simulink model "series_shunt_2a"  (Simulink 7.4)
settings: Solver=ode23tb  StartTime=0.0  StopTime=100e-6  MaxStep=10e-9  RelTol=1e-4
InitFcn:
  | series_shunt_2c;
StopFcn:
  | if ~SPECTRUM_FLAG
  |      %% plot measured sparameters using RFTB
  |     amp=rfdata.data;
  |     amp.Freq=spar(:,1);
  | %%
  |     amp.S_parameters=complex(zeros(2,2,length(amp.Freq)));
  |    if spar(1,6)==1
  |       amp.S_Parameters(1,1,:)=spar(:,2)+1i*spar(:,3);
  |       amp.S_Parameters(2,1,:)=spar(:,4)+1i*spar(:,5);
  |       subplot(2,1,1);
  |       hplot1= smith(amp,'s11')
  |       subplot(2,1,2);
  |       hplot2 = plot(amp,'s21');
  |       axis([amp.Freq(1)/1e6,amp.Freq(end)/1e6,0,20]);
  |    else
  |       amp.S_Parameters(2,2,:)=spar(:,2)+1i*spar(:,3);
  |       amp.S_Parameters(1,2,:)=spar(:,4)+1i*spar(:,5);
  |       subplot(2,1,1);
  |       hplot1= smith(amp,'s22')
  |       subplot(2,1,2);
  |       hplot2 = plot(amp,'s12');
  |    end;
  | end
values from neighbouring files (symbols this model uses):
  Base_Bias = 0.8    [series_shunt_2c.m]
  Beta = 100    [series_shunt_2c.m]
  Cbc = 10e-12    (= 1e-11)    [series_shunt_2c.m]
  Cbe = 250e-12    (= 2.5e-10)    [series_shunt_2c.m]
  ICs = IEs    (= 1e-12)    [series_shunt_2c.m]
  IEs = 1e-12    [series_shunt_2c.m]
  Lpri_1 = 5e-6    (= 5e-06)    [series_shunt_2c.m]
  Lsec_1 = Lpri_1*Tr_1^2    [series_shunt_2c.m]
  M12_1 = K*Tr_1*Lpri_1    [series_shunt_2c.m]
  M13_1 = M12_1    [series_shunt_2c.m]
  M23_1 = K*Lsec_1    [series_shunt_2c.m]
  Rbb = 5    [series_shunt_2c.m]
  Re = (Rl^2)/Rfb    (= 1.52007654004)    [series_shunt_2c.m]
  Rfb = Rl*(1*Av+1)    (= 81.21748272)    [series_shunt_2c.m]
  Rloss = .1    (= 0.1)    [series_shunt_2c.m]
  Vcc = 12    [series_shunt_2c.m]
undefined symbols (not defined in the file or in its folder): Fs, magnitude, One, sided
libraries: powerlib x52, dspindex x12, dspsigops x6, dsparch4 x5, simulink x4, dspbuff3 x4, dspxfrm3 x4, dsparch3 x4, dspsnks4 x3, dspmtrx3 x2
(part 1 of 2)
settings Model: Creator=Dick  LastModifiedBy=Dick

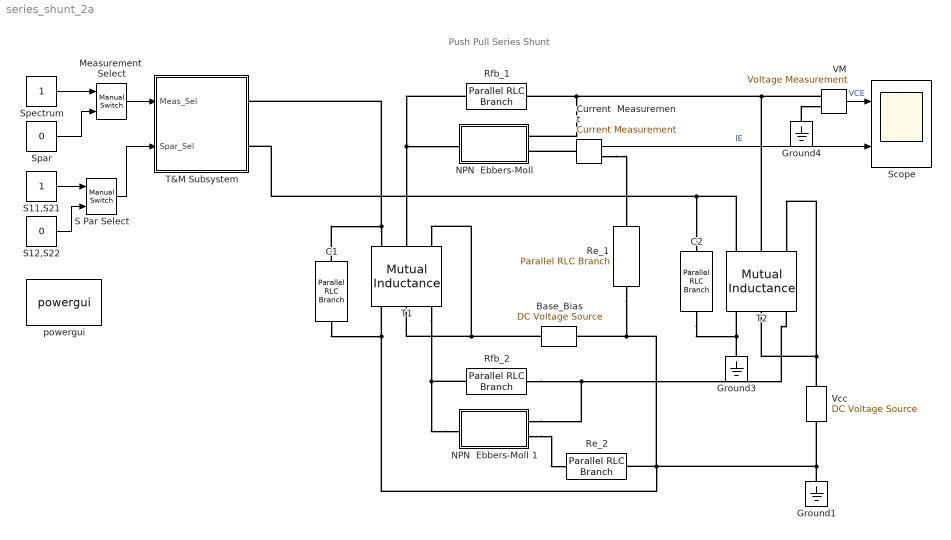
== system series_shunt_2a ==
  note: Push Pull Series Shunt
  Base_Bias : powerlib/Electrical Sources/DC Voltage Source  DialogController=POWERSYS.PowerSysDialog  SystemSampleTime=-1  Amplitude=Base_Bias  Measurements=None
  C1 : powerlib/Elements/Parallel RLC Branch  DialogController=POWERSYS.PowerSysDialog  PhysicalDomain=powersysdomain  SubClassName=unknown  LeftPortType=p1  RightPortType=p1  LConnTagsString=a  RConnTagsString=__new0  BranchType=C  Resistance=1  Inductance=1e-3  SetiL0=off  InitialCurrent=0  Capacitance=2.7e-12  Setx0=off  InitialVoltage=0  Measurements=None
  C2 : powerlib/Elements/Parallel RLC Branch  DialogController=POWERSYS.PowerSysDialog  PhysicalDomain=powersysdomain  SubClassName=unknown  LeftPortType=p1  RightPortType=p1  LConnTagsString=a  RConnTagsString=__new0  BranchType=C  Resistance=1  Inductance=1e-3  SetiL0=off  InitialCurrent=0  Capacitance=27e-12  Setx0=off  InitialVoltage=0  Measurements=None
  Current  Measurement : powerlib/Measurements/Current Measurement  DialogController=POWERSYS.PowerSysDialog  SystemSampleTime=-1  PhasorSimulation=off  OutputType=Complex  PSBequivalent=0
  Ground1 : powerlib/Elements/Ground  DialogController=POWERSYS.PowerSysDialog  PhysicalDomain=powersysdomain  SubClassName=unknown  LeftPortType=p1  RightPortType=p1  LConnTagsString=a
  Ground3 : powerlib/Elements/Ground  DialogController=POWERSYS.PowerSysDialog  PhysicalDomain=powersysdomain  SubClassName=unknown  LeftPortType=p1  RightPortType=p1  LConnTagsString=a
  Ground4 : powerlib/Elements/Ground  DialogController=POWERSYS.PowerSysDialog  PhysicalDomain=powersysdomain  SubClassName=unknown  LeftPortType=p1  RightPortType=p1  LConnTagsString=a
  Measurement  Select : simulink/Signal Routing/Manual Switch  SystemSampleTime=-1  sw=0  action=0  varsize=off
  "NPN  Ebbers-Moll " : Subsystem  mask{Beta=Beta, IEs=IEs, ICs=ICs, Ro=1e5, Cbc=Cbc, Cbe=Cbe, Rbb=Rbb}
      mask init:
      | k = 1.38e-23;
      | q = 1.6e-19;
      | T = 290;
      | Vt = k*T/q;
  NPN  Ebbers-Moll 1 : Subsystem  mask{Beta=Beta, IEs=IEs, ICs=ICs, Ro=1e5, Cbc=Cbc, Cbe=Cbe, Rbb=Rbb}
      mask init:
      | k = 1.38e-23;
      | q = 1.6e-19;
      | T = 290;
      | Vt = k*T/q;
  Re_1 : powerlib/Elements/Parallel RLC Branch  DialogController=POWERSYS.PowerSysDialog  PhysicalDomain=powersysdomain  SubClassName=unknown  LeftPortType=p1  RightPortType=p1  LConnTagsString=a  RConnTagsString=__new0  BranchType=R  Resistance=Re  Inductance=1e-3  SetiL0=off  InitialCurrent=0  Capacitance=1e-6  Setx0=off  InitialVoltage=0  Measurements=None
  Re_2 : powerlib/Elements/Parallel RLC Branch  DialogController=POWERSYS.PowerSysDialog  PhysicalDomain=powersysdomain  SubClassName=unknown  LeftPortType=p1  RightPortType=p1  LConnTagsString=a  RConnTagsString=__new0  BranchType=R  Resistance=Re  Inductance=1e-3  SetiL0=off  InitialCurrent=0  Capacitance=1e-6  Setx0=off  InitialVoltage=0  Measurements=None
  Rfb_1 : powerlib/Elements/Parallel RLC Branch  DialogController=POWERSYS.PowerSysDialog  PhysicalDomain=powersysdomain  SubClassName=unknown  LeftPortType=p1  RightPortType=p1  LConnTagsString=a  RConnTagsString=__new0  BranchType=R  Resistance=Rfb  Inductance=1e-3  SetiL0=off  InitialCurrent=0  Capacitance=1e-6  Setx0=off  InitialVoltage=0  Measurements=None
  Rfb_2 : powerlib/Elements/Parallel RLC Branch  DialogController=POWERSYS.PowerSysDialog  PhysicalDomain=powersysdomain  SubClassName=unknown  LeftPortType=p1  RightPortType=p1  LConnTagsString=a  RConnTagsString=__new0  BranchType=R  Resistance=Rfb  Inductance=1e-3  SetiL0=off  InitialCurrent=0  Capacitance=1e-6  Setx0=off  InitialVoltage=0  Measurements=None
  S Par Select : simulink/Signal Routing/Manual Switch  SystemSampleTime=-1  sw=1  action=0  varsize=off
  S11,S21 : Constant  OutDataType=fixdt(1, 16)  OutScaling=2^0
  S12,S22 : Constant  Value=0  OutDataType=fixdt(1, 16)  OutScaling=2^0
  Scope : Scope  NumInputPorts=2
      settings: TimeRange=5e-006  YMin=-17.5~-0.1  YMax=17.5~1.5
  Spar : Constant  Value=0  OutDataTypeMode=boolean  OutDataType=fixdt(1, 16)  OutScaling=2^0  OutDataTypeStr=boolean
  Spectrum : Constant  OutDataTypeMode=boolean  OutDataType=fixdt(1, 16)  OutScaling=2^0  OutDataTypeStr=boolean
  T&M Subsystem : Subsystem
  T1 : powerlib/Elements/Mutual Inductance  DialogController=POWERSYS.PowerSysDialog  PhysicalDomain=powersysdomain  SubClassName=unknown  LeftPortType=p1  RightPortType=p1  LConnTagsString=a|b|c  RConnTagsString=A|B|C  TypeOfMutual=Generalized mutual inductance  NumberOfWindings=3  SelfImpedance1=[1.1 1.1e-03]  SelfImpedance2=[ 1.1 1.1e-03]  ThreeWindings=on  SelfImpedance3=[ 1.1 1.1e-03]  MutualImpedance=[1.0 1.0e-03]  InductanceMatrix=[Lpri_1 M12_1 M13_1; M12_1 Lsec_1 M23_1; M13_1 M23_1 Lsec_1];  ResistanceMatrix="[1  0 0 ; 0 1 0 ; 0 0 1]*Rloss;"  Measurements=None
      settings: AttributesFormatString=\n
  T2 : powerlib/Elements/Mutual Inductance  DialogController=POWERSYS.PowerSysDialog  PhysicalDomain=powersysdomain  SubClassName=unknown  LeftPortType=p1  RightPortType=p1  LConnTagsString=a|b|c  RConnTagsString=A|B|C  TypeOfMutual=Generalized mutual inductance  NumberOfWindings=3  SelfImpedance1=[1.1 1.1e-03]  SelfImpedance2=[ 1.1 1.1e-03]  ThreeWindings=on  SelfImpedance3=[ 1.1 1.1e-03]  MutualImpedance=[1.0 1.0e-03]  InductanceMatrix=[Lpri_1 M12_1 M13_1; M12_1 Lsec_1 M23_1; M13_1 M23_1 Lsec_1];  ResistanceMatrix="[1  0 0 ; 0 1 0 ; 0 0 1]*Rloss;"  Measurements=None
      settings: AttributesFormatString=\n
  VM : powerlib/Measurements/Voltage Measurement  DialogController=POWERSYS.PowerSysDialog  SystemSampleTime=-1  PhasorSimulation=off  OutputType=Complex  PSBequivalent=0
  Vcc : powerlib/Electrical Sources/DC Voltage Source  DialogController=POWERSYS.PowerSysDialog  SystemSampleTime=-1  Amplitude=Vcc  Measurements=None
  powergui : powerlib/powergui  Priority=1  SystemSampleTime=-1  SimulationMode=Continuous  SampleTime=50e-6  frequency=60  SPID=off  DisableSnubberDevices=off  DisableRonSwitches=off  DisableVfSwitches=off  SwTol=0  Interpol=off  frequencyindice=0  echomessages=off  HookPort=off  DisplayEquations=off  FunctionMessages=off  EnableUseOfTLC=off  x0status=blocks  RestoreLinks=warning  Frange=[0:2:500]  Ylog=off  Xlog=on  ShowGrid=off  save=off  variable=ZData  ZoomFFT=on  StartTime=0.0  cycles=1  DisplayStyle=1  fundamental=60  FreqAxis=off  MaxFrequency=1000  frequencyindicesteady=1  RmsSteady=1  display=off  Ts=0  methode=off
  wires:
  Measurement  Select/1 -> T&M Subsystem/1(Meas_Sel)
  Spar/1 -> Measurement  Select/2
  Spectrum/1 -> Measurement  Select/1
  S Par Select/1 -> T&M Subsystem/2(Spar_Sel)
  S11,S21/1 -> S Par Select/1
  S12,S22/1 -> S Par Select/2
  VM/1 -> Scope/1  "VCE"
  Current  Measurement/1 -> Scope/2  "IE"
  connections:
  VM/LConn1 -- Rfb_1/LConn1 -- "NPN  Ebbers-Moll "/RConn1 -- T2/RConn2
  Rfb_1/RConn1 -- T1/RConn2 -- "NPN  Ebbers-Moll "/LConn1
  Base_Bias/LConn1 -- Re_1/RConn1 -- Re_2/LConn1 -- Ground1/LConn1 -- Vcc/LConn1 -- T1/LConn1 -- C1/RConn1
  T1/RConn1 -- C1/LConn1 -- T&M Subsystem/RConn1
  T2/RConn1 -- T&M Subsystem/RConn2 -- C2/LConn1
  Current  Measurement/LConn1 -- "NPN  Ebbers-Moll "/RConn2
  Current  Measurement/RConn1 -- Re_1/LConn1
  Vcc/RConn1 -- T2/RConn3 -- T2/LConn2
  Ground3/LConn1 -- T2/LConn1 -- C2/RConn1
  T1/LConn2 -- Base_Bias/RConn1 -- T1/RConn3
  NPN  Ebbers-Moll 1/LConn1 -- T1/LConn3 -- Rfb_2/RConn1
  Rfb_2/LConn1 -- T2/LConn3 -- NPN  Ebbers-Moll 1/RConn1
  Ground4/LConn1 -- VM/LConn2
  NPN  Ebbers-Moll 1/RConn2 -- Re_2/RConn1

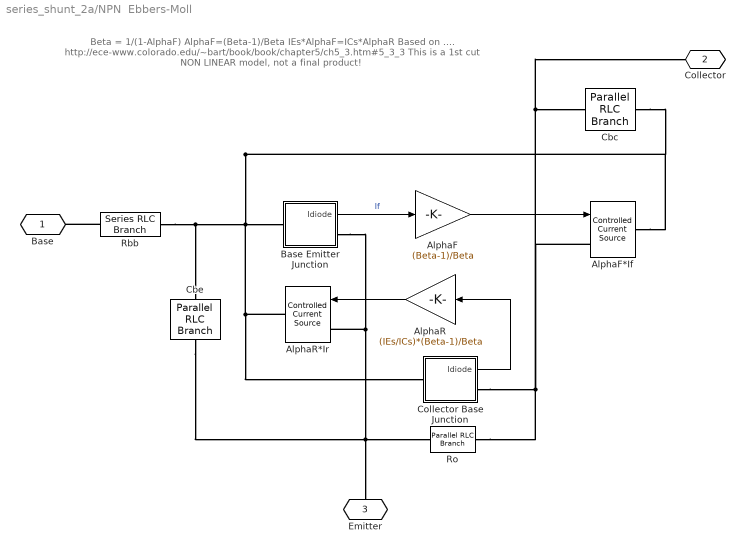
== system series_shunt_2a/NPN  Ebbers-Moll  ==
  note: Beta = 1/(1-AlphaF)
      | AlphaF=(Beta-1)/Beta
      | IEs*AlphaF=ICs*AlphaR
      |
      | Based on ....
      | http://ece-www.colorado.edu/~bart/book/book/chapter5/ch5_3.htm#5_3_3
      |
      | This is a 1st cut NON LINEAR model, not a final product!
  AlphaF : Gain  Gain=(Beta-1)/Beta  ParameterDataType=sfix(16)  ParameterScaling=2^0  OutDataType=sfix(16)  OutScaling=2^0
  AlphaF*If : powerlib/Electrical Sources/Controlled Current Source  Description=source block  DialogController=POWERSYS.PowerSysDialog  SystemSampleTime=-1  Initialize=off  Source_Type=AC  Amplitude=-0.025  Phase=0  Frequency=0  Measurements=None
      settings: AttributesFormatString=\n
  AlphaR : Gain  Gain=(IEs/ICs)*(Beta-1)/Beta  ParameterDataType=sfix(16)  ParameterScaling=2^0  OutDataType=sfix(16)  OutScaling=2^0
  AlphaR*Ir : powerlib/Electrical Sources/Controlled Current Source  Description=source block  DialogController=POWERSYS.PowerSysDialog  SystemSampleTime=-1  Initialize=off  Source_Type=AC  Amplitude=-0.025  Phase=0  Frequency=0  Measurements=None
      settings: AttributesFormatString=\n
  Base Emitter Junction : Subsystem  AncestorBlock=simcircuits_library_1/diode  mask{Is=IEs}
      mask prompts: Is "Saturation Current"
      mask Display: plot(-140,-140,150,140,2*[30,30,59,30,30,0]-75,(2*[71,50,72,92,71,71]-92),2*[59,59]-75,(2*[50,93]-92),[116,59]-16,(2*[71,71]-90));
  Cbc : powerlib/Elements/Parallel RLC Branch  DialogController=POWERSYS.PowerSysDialog  PhysicalDomain=powersysdomain  SubClassName=unknown  LeftPortType=p1  RightPortType=p1  LConnTagsString=a  RConnTagsString=__new0  BranchType=C  Resistance=1.0  Inductance=1.0  SetiL0=off  InitialCurrent=0  Capacitance=Cbc  Setx0=off  InitialVoltage=0  Measurements=None
  Cbe : powerlib/Elements/Parallel RLC Branch  DialogController=POWERSYS.PowerSysDialog  PhysicalDomain=powersysdomain  SubClassName=unknown  LeftPortType=p1  RightPortType=p1  LConnTagsString=a  RConnTagsString=__new0  BranchType=C  Resistance=1.0  Inductance=1.0  SetiL0=off  InitialCurrent=0  Capacitance=Cbe  Setx0=off  InitialVoltage=0  Measurements=None
  Collector Base Junction : Subsystem  AncestorBlock=simcircuits_library_1/diode  mask{Is=ICs}
      mask prompts: Is "Saturation Current"
      mask Display: plot(-140,-140,150,140,2*[30,30,59,30,30,0]-75,(2*[71,50,72,92,71,71]-92),2*[59,59]-75,(2*[50,93]-92),[116,59]-16,(2*[71,71]-90));
  Rbb : powerlib/Elements/Series RLC Branch  DialogController=POWERSYS.PowerSysDialog  PhysicalDomain=powersysdomain  SubClassName=unknown  LeftPortType=p1  RightPortType=p1  LConnTagsString=__new0  RConnTagsString=__new0  BranchType=R  Resistance=Rbb  Inductance=1.0  SetiL0=off  InitialCurrent=0  Capacitance=1.0  Setx0=off  InitialVoltage=0  Measurements=None
  Ro : powerlib/Elements/Parallel RLC Branch  DialogController=POWERSYS.PowerSysDialog  PhysicalDomain=powersysdomain  SubClassName=unknown  LeftPortType=p1  RightPortType=p1  LConnTagsString=a  RConnTagsString=__new0  BranchType=R  Resistance=Ro  Inductance=1.0  SetiL0=off  InitialCurrent=0  Capacitance=1.0  Setx0=off  InitialVoltage=0  Measurements=None
  Base : PMIOPort  Port=1  Side=Left
  Collector : PMIOPort  Port=2  Side=Right
  Emitter : PMIOPort  Port=3  Side=Right
  wires:
  Base Emitter Junction/1(Idiode) -> AlphaF/1  "If"
  AlphaF/1 -> AlphaF*If/1
  Collector Base Junction/1(Idiode) -> AlphaR/1
  AlphaR/1 -> AlphaR*Ir/1
  connections:
  Rbb/RConn1 -- Cbe/LConn1 -- Base Emitter Junction/LConn1 -- AlphaF*If/RConn1 -- Cbc/RConn1 -- AlphaR*Ir/RConn1 -- Collector Base Junction/LConn1
  AlphaR*Ir/LConn1 -- Emitter/RConn1 -- Cbe/RConn1 -- Ro/LConn1 -- Base Emitter Junction/RConn1
  AlphaF*If/LConn1 -- Collector/RConn1 -- Cbc/LConn1 -- Collector Base Junction/RConn1 -- Ro/RConn1
  Rbb/LConn1 -- Base/RConn1

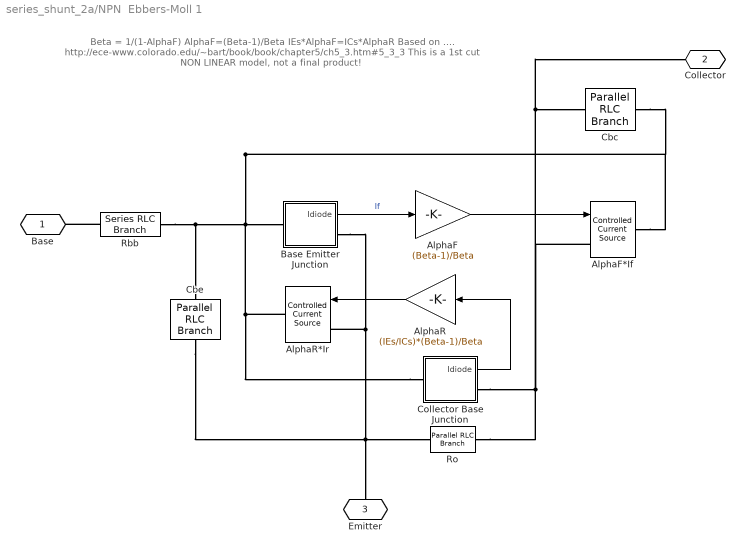
== system series_shunt_2a/NPN  Ebbers-Moll 1 ==
  note: Beta = 1/(1-AlphaF)
      | AlphaF=(Beta-1)/Beta
      | IEs*AlphaF=ICs*AlphaR
      |
      | Based on ....
      | http://ece-www.colorado.edu/~bart/book/book/chapter5/ch5_3.htm#5_3_3
      |
      | This is a 1st cut NON LINEAR model, not a final product!
  AlphaF : Gain  Gain=(Beta-1)/Beta  ParameterDataType=sfix(16)  ParameterScaling=2^0  OutDataType=sfix(16)  OutScaling=2^0
  AlphaF*If : powerlib/Electrical Sources/Controlled Current Source  Description=source block  DialogController=POWERSYS.PowerSysDialog  SystemSampleTime=-1  Initialize=off  Source_Type=AC  Amplitude=-0.025  Phase=0  Frequency=0  Measurements=None
      settings: AttributesFormatString=\n
  AlphaR : Gain  Gain=(IEs/ICs)*(Beta-1)/Beta  ParameterDataType=sfix(16)  ParameterScaling=2^0  OutDataType=sfix(16)  OutScaling=2^0
  AlphaR*Ir : powerlib/Electrical Sources/Controlled Current Source  Description=source block  DialogController=POWERSYS.PowerSysDialog  SystemSampleTime=-1  Initialize=off  Source_Type=AC  Amplitude=-0.025  Phase=0  Frequency=0  Measurements=None
      settings: AttributesFormatString=\n
  Base Emitter Junction : Subsystem  AncestorBlock=simcircuits_library_1/diode  mask{Is=IEs}
      mask prompts: Is "Saturation Current"
      mask Display: plot(-140,-140,150,140,2*[30,30,59,30,30,0]-75,(2*[71,50,72,92,71,71]-92),2*[59,59]-75,(2*[50,93]-92),[116,59]-16,(2*[71,71]-90));
  Cbc : powerlib/Elements/Parallel RLC Branch  DialogController=POWERSYS.PowerSysDialog  PhysicalDomain=powersysdomain  SubClassName=unknown  LeftPortType=p1  RightPortType=p1  LConnTagsString=a  RConnTagsString=__new0  BranchType=C  Resistance=1.0  Inductance=1.0  SetiL0=off  InitialCurrent=0  Capacitance=Cbc  Setx0=off  InitialVoltage=0  Measurements=None
  Cbe : powerlib/Elements/Parallel RLC Branch  DialogController=POWERSYS.PowerSysDialog  PhysicalDomain=powersysdomain  SubClassName=unknown  LeftPortType=p1  RightPortType=p1  LConnTagsString=a  RConnTagsString=__new0  BranchType=C  Resistance=1.0  Inductance=1.0  SetiL0=off  InitialCurrent=0  Capacitance=Cbe  Setx0=off  InitialVoltage=0  Measurements=None
  Collector Base Junction : Subsystem  AncestorBlock=simcircuits_library_1/diode  mask{Is=ICs}
      mask prompts: Is "Saturation Current"
      mask Display: plot(-140,-140,150,140,2*[30,30,59,30,30,0]-75,(2*[71,50,72,92,71,71]-92),2*[59,59]-75,(2*[50,93]-92),[116,59]-16,(2*[71,71]-90));
  Rbb : powerlib/Elements/Series RLC Branch  DialogController=POWERSYS.PowerSysDialog  PhysicalDomain=powersysdomain  SubClassName=unknown  LeftPortType=p1  RightPortType=p1  LConnTagsString=__new0  RConnTagsString=__new0  BranchType=R  Resistance=Rbb  Inductance=1.0  SetiL0=off  InitialCurrent=0  Capacitance=1.0  Setx0=off  InitialVoltage=0  Measurements=None
  Ro : powerlib/Elements/Parallel RLC Branch  DialogController=POWERSYS.PowerSysDialog  PhysicalDomain=powersysdomain  SubClassName=unknown  LeftPortType=p1  RightPortType=p1  LConnTagsString=a  RConnTagsString=__new0  BranchType=R  Resistance=Ro  Inductance=1.0  SetiL0=off  InitialCurrent=0  Capacitance=1.0  Setx0=off  InitialVoltage=0  Measurements=None
  Base : PMIOPort  Port=1  Side=Left
  Collector : PMIOPort  Port=2  Side=Right
  Emitter : PMIOPort  Port=3  Side=Right
  wires:
  AlphaR/1 -> AlphaR*Ir/1
  Collector Base Junction/1(Idiode) -> AlphaR/1
  AlphaF/1 -> AlphaF*If/1
  Base Emitter Junction/1(Idiode) -> AlphaF/1  "If"
  connections:
  Rbb/LConn1 -- Base/RConn1
  Ro/RConn1 -- Collector Base Junction/RConn1 -- Cbc/LConn1 -- Collector/RConn1 -- AlphaF*If/LConn1
  Base Emitter Junction/RConn1 -- Ro/LConn1 -- Cbe/RConn1 -- Emitter/RConn1 -- AlphaR*Ir/LConn1
  Collector Base Junction/LConn1 -- AlphaR*Ir/RConn1 -- Cbc/RConn1 -- AlphaF*If/RConn1 -- Base Emitter Junction/LConn1 -- Cbe/LConn1 -- Rbb/RConn1

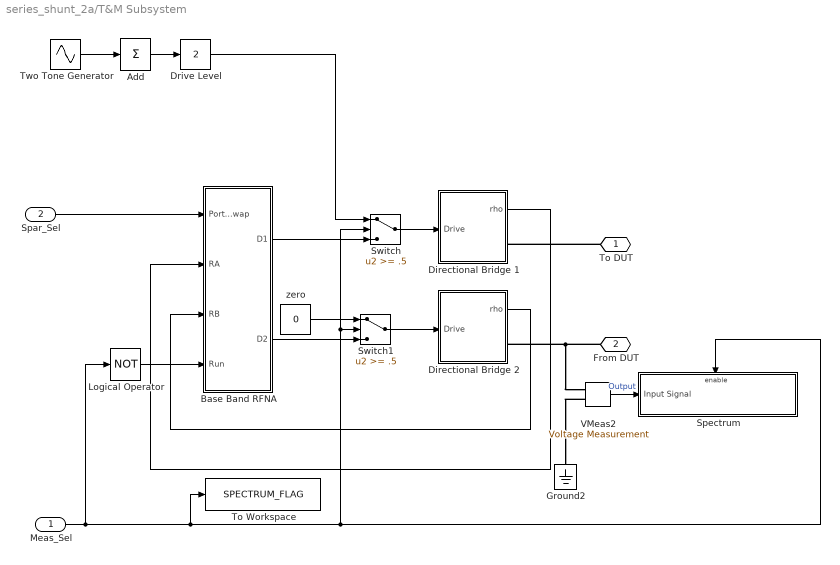
== system series_shunt_2a/T&M Subsystem ==
  Meas_Sel : Inport  OutDataType=fixdt(1, 16)  OutScaling=2^0
  Spar_Sel : Inport  Port=2  OutDataType=fixdt(1, 16)  OutScaling=2^0
  Add : Sum  Inputs=+  OutDataType=fixdt(1, 16)  OutScaling=2^-10
  Base Band RFNA : Subsystem  Description=Spectrum Analyzer  mask{BW=30e6, Frame_Size=256}
      mask prompts: BW "Bandwidth"; Frame_Size "FFT SIze (256,512,1024 etc)"
  Directional Bridge 1 : Subsystem  mask{Zo=50}
      mask prompts: Zo "Zo="
  Directional Bridge 2 : Subsystem  mask{Zo=50}
      mask prompts: Zo "Zo="
  Drive Level : simulink/Math Operations/Slider Gain  SystemSampleTime=-1  low=0.2  gain=2  high=4
  Ground2 : powerlib/Elements/Ground  DialogController=POWERSYS.PowerSysDialog  PhysicalDomain=powersysdomain  SubClassName=unknown  LeftPortType=p1  RightPortType=p1  LConnTagsString=a
  Logical Operator : Logic  Operator=NOT  AllPortsSameDT=off  OutDataTypeMode=boolean  LogicDataType=fixdt(0, 8)  OutDataTypeStr=boolean
  Spectrum : Subsystem  Description=Spectrum Analyzer  mask{BW=30e6, Zo=50}
      mask prompts: BW "Bandwidth"; Zo "Load Zo"
      mask Display: fprintf('Baseband Spectrum Analyzer \n  BW=%7.2f MHz', BW/1e6)
  Switch : Switch  Threshold=.5  OutDataType=fixdt(1, 16)  OutScaling=2^0
  Switch1 : Switch  Threshold=.5  OutDataType=fixdt(1, 16)  OutScaling=2^0
  To Workspace : ToWorkspace  VariableName=SPECTRUM_FLAG  SampleTime=-1  SaveFormat=Array
      settings: MaxDataPoints=1
  Two Tone Generator : Sin  Amplitude=2*sqrt(2)  Bias=0  Frequency=[10e6 12e6]*2*pi  Phase=0  Samples=10  SampleTime=0  Offset=0
  VMeas2 : powerlib/Measurements/Voltage Measurement  DialogController=POWERSYS.PowerSysDialog  SystemSampleTime=-1  PhasorSimulation=off  OutputType=Complex  PSBequivalent=0
  zero : Constant  Value=0  OutDataTypeMode=boolean  OutDataType=fixdt(1, 16)  OutScaling=2^0  OutDataTypeStr=boolean
  To DUT : PMIOPort  Port=1  Side=Right
  From DUT : PMIOPort  Port=2  Side=Right
  wires:
  Two Tone Generator/1 -> Add/1
  Directional Bridge 1/1(rho) -> Base Band RFNA/2(RA)
  Directional Bridge 2/1(rho) -> Base Band RFNA/3(RB)
  VMeas2/1 -> Spectrum/1(Input Signal)  "Output"
  Base Band RFNA/1(D1) -> Switch/3
  Switch/1 -> Directional Bridge 1/1(Drive)
  Add/1 -> Drive Level/1
  Switch1/1 -> Directional Bridge 2/1(Drive)
  Base Band RFNA/2(D2) -> Switch1/3
  zero/1 -> Switch1/1
  Logical Operator/1 -> Base Band RFNA/4(Run)
  Meas_Sel/1 -> Logical Operator/1, Switch1/2, Switch/2, Spectrum/Enable, To Workspace/1
  Spar_Sel/1 -> Base Band RFNA/1(Port Swap)
  Drive Level/1 -> Switch/1
  connections:
  From DUT/RConn1 -- Directional Bridge 2/RConn1 -- VMeas2/LConn1
  VMeas2/LConn2 -- Ground2/LConn1
  To DUT/RConn1 -- Directional Bridge 1/RConn1

== system series_shunt_2a/NPN  Ebbers-Moll /Base Emitter Junction ==
  Diode Equation : Fcn  Expr="Is* (exp(u /.025)  -1  );  % ideal diode equation @ room temp"
  "Vf " : powerlib/Measurements/Voltage Measurement  Tag=PoWeRsYsTeMmEaSuReMeNt  DialogController=POWERSYS.PowerSysDialog  SystemSampleTime=-1  PhasorSimulation=off  OutputType=Magnitude  PSBequivalent=0
  ik1 : powerlib/Electrical Sources/Controlled Current Source  Description=source block  DialogController=POWERSYS.PowerSysDialog  SystemSampleTime=-1  Initialize=on  Source_Type=AC  Amplitude=0  Phase=0  Frequency=0  Measurements=None
      settings: AttributesFormatString=\n
  Anode : PMIOPort  Tag=PMCPort  Port=1  Side=Left
  "cathode " : PMIOPort  Tag=PMCPort  Port=2  Side=Right
  Idiode : Outport  OutDataType=sfix(16)  OutScaling=2^0
  wires:
  "Vf "/1 -> Diode Equation/1
  Diode Equation/1 -> ik1/1, Idiode/1
  connections:
  "Vf "/LConn1 -- Anode/RConn1 -- ik1/LConn1
  "Vf "/LConn2 -- "cathode "/RConn1 -- ik1/RConn1

== system series_shunt_2a/NPN  Ebbers-Moll /Collector Base Junction ==
  Diode Equation : Fcn  Expr="Is* (exp(u /.025)  -1  );  % ideal diode equation @ room temp"
  "Vf " : powerlib/Measurements/Voltage Measurement  Tag=PoWeRsYsTeMmEaSuReMeNt  DialogController=POWERSYS.PowerSysDialog  SystemSampleTime=-1  PhasorSimulation=off  OutputType=Magnitude  PSBequivalent=0
  ik1 : powerlib/Electrical Sources/Controlled Current Source  Description=source block  DialogController=POWERSYS.PowerSysDialog  SystemSampleTime=-1  Initialize=on  Source_Type=AC  Amplitude=0  Phase=0  Frequency=0  Measurements=None
      settings: AttributesFormatString=\n
  Anode : PMIOPort  Tag=PMCPort  Port=1  Side=Left
  "cathode " : PMIOPort  Tag=PMCPort  Port=2  Side=Right
  Idiode : Outport  OutDataType=sfix(16)  OutScaling=2^0
  wires:
  Diode Equation/1 -> Idiode/1, ik1/1
  "Vf "/1 -> Diode Equation/1
  connections:
  ik1/RConn1 -- "cathode "/RConn1 -- "Vf "/LConn2
  ik1/LConn1 -- Anode/RConn1 -- "Vf "/LConn1

== system series_shunt_2a/NPN  Ebbers-Moll 1/Base Emitter Junction ==
  Diode Equation : Fcn  Expr="Is* (exp(u /.025)  -1  );  % ideal diode equation @ room temp"
  "Vf " : powerlib/Measurements/Voltage Measurement  Tag=PoWeRsYsTeMmEaSuReMeNt  DialogController=POWERSYS.PowerSysDialog  SystemSampleTime=-1  PhasorSimulation=off  OutputType=Magnitude  PSBequivalent=0
  ik1 : powerlib/Electrical Sources/Controlled Current Source  Description=source block  DialogController=POWERSYS.PowerSysDialog  SystemSampleTime=-1  Initialize=on  Source_Type=AC  Amplitude=0  Phase=0  Frequency=0  Measurements=None
      settings: AttributesFormatString=\n
  Anode : PMIOPort  Tag=PMCPort  Port=1  Side=Left
  "cathode " : PMIOPort  Tag=PMCPort  Port=2  Side=Right
  Idiode : Outport  OutDataType=sfix(16)  OutScaling=2^0
  wires:
  Diode Equation/1 -> Idiode/1, ik1/1
  "Vf "/1 -> Diode Equation/1
  connections:
  ik1/RConn1 -- "cathode "/RConn1 -- "Vf "/LConn2
  ik1/LConn1 -- Anode/RConn1 -- "Vf "/LConn1

== system series_shunt_2a/NPN  Ebbers-Moll 1/Collector Base Junction ==
  Diode Equation : Fcn  Expr="Is* (exp(u /.025)  -1  );  % ideal diode equation @ room temp"
  "Vf " : powerlib/Measurements/Voltage Measurement  Tag=PoWeRsYsTeMmEaSuReMeNt  DialogController=POWERSYS.PowerSysDialog  SystemSampleTime=-1  PhasorSimulation=off  OutputType=Magnitude  PSBequivalent=0
  ik1 : powerlib/Electrical Sources/Controlled Current Source  Description=source block  DialogController=POWERSYS.PowerSysDialog  SystemSampleTime=-1  Initialize=on  Source_Type=AC  Amplitude=0  Phase=0  Frequency=0  Measurements=None
      settings: AttributesFormatString=\n
  Anode : PMIOPort  Tag=PMCPort  Port=1  Side=Left
  "cathode " : PMIOPort  Tag=PMCPort  Port=2  Side=Right
  Idiode : Outport  OutDataType=sfix(16)  OutScaling=2^0
  wires:
  "Vf "/1 -> Diode Equation/1
  Diode Equation/1 -> ik1/1, Idiode/1
  connections:
  "Vf "/LConn1 -- Anode/RConn1 -- ik1/LConn1
  "Vf "/LConn2 -- "cathode "/RConn1 -- ik1/RConn1

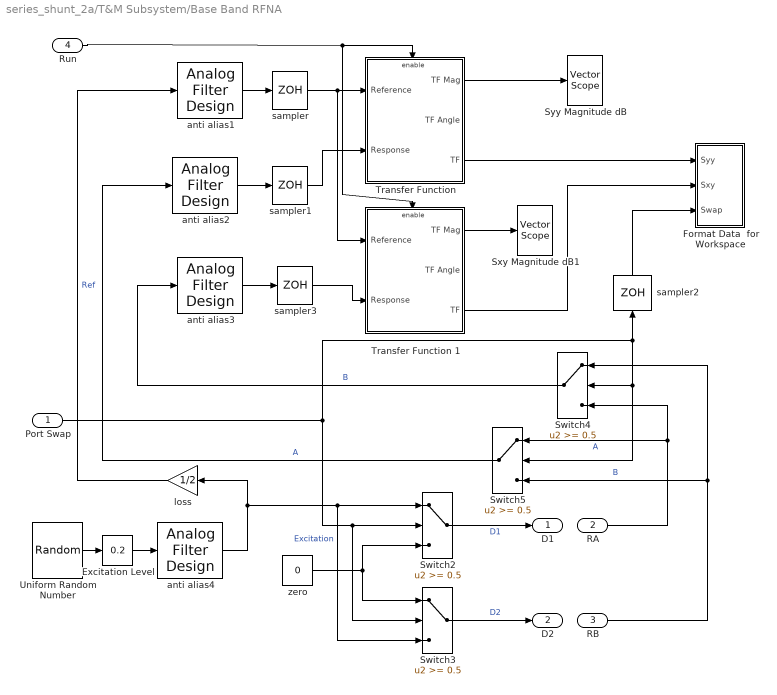
== system series_shunt_2a/T&M Subsystem/Base Band RFNA ==
  Port Swap : Inport  OutDataType=sfix(16)  OutScaling=2^0
  RA : Inport  Port=2  OutDataType=fixdt(1, 16)  OutScaling=2^0
  RB : Inport  Port=3  OutDataType=fixdt(1, 16)  OutScaling=2^0
  Run : Inport  Port=4  OutDataType=sfix(16)  OutScaling=2^0
  Excitation Level : simulink/Math Operations/Slider Gain  SystemSampleTime=-1  low=0  gain=0.2  high=1
  Format Data  for Workspace : Subsystem
  Switch{2..5} (4 alike) : Switch  Threshold=0.5  SaturateOnIntegerOverflow=on
  Sxy Magnitude dB1 : dspsnks4/Vector Scope  DialogController=dspdialog.VectorScope  DialogControllerArgs=DataTag0  ScopeProperties=on  Domain=Frequency  HorizSpan=1  DisplayProperties=off  AxisGrid=on  Memory=off  FrameNumber=on  AxisLegend=off  AxisZoom=off  OpenScopeAtSimStart=on  OpenScopeImmediately=off  FigPos=[414 33 372 236]  AxisProperties=off  XUnits=Hertz  XRange=[0...Fs/2]  InheritXIncr=on  XIncr=2*Fs  XLabel=Time  XLimit=Auto  XMin=0  XMax=1  XStart=0  YUnits=dB  YLabel=dB  LineProperties=off  LineColors=[1 0 0]|[1 0 0]  XAxisParamsVer=6.9
      settings: YMin=0  YMax=25
  Syy Magnitude dB : dspsnks4/Vector Scope  DialogController=dspdialog.VectorScope  DialogControllerArgs=DataTag1  ScopeProperties=on  Domain=Frequency  HorizSpan=1  DisplayProperties=off  AxisGrid=on  Memory=off  FrameNumber=on  AxisLegend=off  AxisZoom=off  OpenScopeAtSimStart=on  OpenScopeImmediately=off  FigPos=[32 34 372 236]  AxisProperties=off  XUnits=Hertz  XRange=[0...Fs/2]  InheritXIncr=on  XIncr=2*Fs  XLabel=Time  XLimit=Auto  XMin=0  XMax=128000000  XStart=0  YUnits=dB  YLabel=dB  LineProperties=off  LineColors=[1 0 0]|[1 0 0]  XAxisParamsVer=6.9
      settings: YMin=-40  YMax=0
  "Transfer Function " : Subsystem  mask{NFFT=Frame_Size, Navg=100, pcnt=100, unwrap_flag=on}
      mask prompts: NFFT "FFT length (power of 2):"; Navg "Spectral Averaging Factor (>=1):"; pcnt "Percentage of  Alias Free Data  (<=100)"; unwrap_flag "Unwrap Phase"
      mask Display: disp('Transfer Function \n Estimation (v2.0) ')
  Transfer Function 1 : Subsystem  mask{NFFT=Frame_Size, Navg=100, pcnt=100, unwrap_flag=on}
      mask prompts: NFFT "FFT length (power of 2):"; Navg "Spectral Averaging Factor (>=1):"; pcnt "Percentage of  Alias Free Data  (<=100)"; unwrap_flag "Unwrap Phase"
      mask Display: disp('Transfer Function \n Estimation (v2.0) ')
  Uniform Random Number : UniformRandomNumber  SampleTime=1/(2.56*BW)
  anti alias{1..4} (4 alike) : dsparch4/Analog Filter Design  method=Elliptic  filttype=Lowpass  N=8  Wlo=BW*2*pi  Whi=80  Rp=2  Rs=100
  loss : Gain  Gain=1/2  ParameterDataType=sfix(16)  ParameterScaling=2^0  OutDataType=sfix(16)  OutScaling=2^0  SaturateOnIntegerOverflow=on  OutDataTypeStr=Inherit: Same as input  ParamDataTypeStr=Inherit: Same as input
  sampler : ZeroOrderHold  SampleTime=1/(2.56*BW)
  sampler1 : ZeroOrderHold  SampleTime=1/(2.56*BW)
  sampler2 : ZeroOrderHold  SampleTime=256/(2.56*BW)
  sampler3 : ZeroOrderHold  SampleTime=1/(2.56*BW)
  zero : Constant  Value=0  OutDataType=sfix(16)  OutScaling=2^0
  D1 : Outport  OutDataType=fixdt(1, 16)  OutScaling=2^0
  D2 : Outport  Port=2  OutDataType=fixdt(1, 16)  OutScaling=2^0
  wires:
  sampler/1 -> "Transfer Function "/1(Reference), Transfer Function 1/1(Reference)
  anti alias1/1 -> sampler/1
  anti alias2/1 -> sampler1/1
  Uniform Random Number/1 -> Excitation Level/1
  anti alias3/1 -> sampler3/1
  sampler3/1 -> Transfer Function 1/2(Response)
  anti alias4/1 -> loss/1, Switch3/3, Switch2/1  "Excitation"
  loss/1 -> anti alias1/1  "Ref"
  Port Swap/1 -> Switch3/2, Switch2/2, Switch4/2, Switch5/2, sampler2/1
  zero/1 -> Switch2/3, Switch3/1
  Switch2/1 -> D1/1  "D1"
  Switch3/1 -> D2/1  "D2"
  Switch5/1 -> anti alias2/1  "A"
  Switch4/1 -> anti alias3/1  "B"
  RB/1 -> Switch5/3, Switch4/1  "B"
  sampler1/1 -> "Transfer Function "/2(Response)
  "Transfer Function "/1(TF Mag) -> Syy Magnitude dB/1
  Transfer Function 1/3("TF ") -> Format Data  for Workspace/2(Sxy)
  Transfer Function 1/1(TF Mag) -> Sxy Magnitude dB1/1
  "Transfer Function "/3("TF ") -> Format Data  for Workspace/1(Syy)
  sampler2/1 -> Format Data  for Workspace/3(Swap)
  RA/1 -> Switch4/3, Switch5/1  "A"
  Run/1 -> "Transfer Function "/Enable, Transfer Function 1/Enable
  Excitation Level/1 -> anti alias4/1

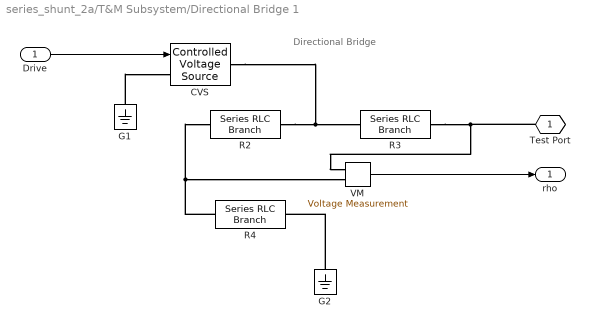
== system series_shunt_2a/T&M Subsystem/Directional Bridge 1 ==
  note: Directional Bridge
  Drive : Inport  OutDataType=sfix(16)  OutScaling=2^0
  CVS : powerlib/Electrical Sources/Controlled Voltage Source  Description=source block  DialogController=POWERSYS.PowerSysDialog  SystemSampleTime=-1  Initialize=off  Source_Type=AC  Amplitude=0  Phase=0  Frequency=0  Measurements=None
      settings: AttributesFormatString=\n
  G1 : powerlib/Elements/Ground  DialogController=POWERSYS.PowerSysDialog  PhysicalDomain=powersysdomain  SubClassName=unknown  LeftPortType=p1  RightPortType=p1  LConnTagsString=a
  G2 : powerlib/Elements/Ground  DialogController=POWERSYS.PowerSysDialog  PhysicalDomain=powersysdomain  SubClassName=unknown  LeftPortType=p1  RightPortType=p1  LConnTagsString=a
  R2 : powerlib/Elements/Series RLC Branch  DialogController=POWERSYS.PowerSysDialog  PhysicalDomain=powersysdomain  SubClassName=unknown  LeftPortType=p1  RightPortType=p1  LConnTagsString=__new0  RConnTagsString=__new0  BranchType=R  Resistance=Zo  Inductance=1.0  SetiL0=off  InitialCurrent=0  Capacitance=1.0  Setx0=off  InitialVoltage=0  Measurements=None
  R3 : powerlib/Elements/Series RLC Branch  DialogController=POWERSYS.PowerSysDialog  PhysicalDomain=powersysdomain  SubClassName=unknown  LeftPortType=p1  RightPortType=p1  LConnTagsString=__new0  RConnTagsString=__new0  BranchType=R  Resistance=Zo  Inductance=1.0  SetiL0=off  InitialCurrent=0  Capacitance=1.0  Setx0=off  InitialVoltage=0  Measurements=None
  R4 : powerlib/Elements/Series RLC Branch  DialogController=POWERSYS.PowerSysDialog  PhysicalDomain=powersysdomain  SubClassName=unknown  LeftPortType=p1  RightPortType=p1  LConnTagsString=__new0  RConnTagsString=__new0  BranchType=R  Resistance=Zo  Inductance=1.0  SetiL0=off  InitialCurrent=0  Capacitance=1.0  Setx0=off  InitialVoltage=0  Measurements=None
  VM : powerlib/Measurements/Voltage Measurement  Tag=PoWeRsYsTeMmEaSuReMeNt  DialogController=POWERSYS.PowerSysDialog  SystemSampleTime=-1  PhasorSimulation=off  OutputType=Magnitude  PSBequivalent=0
  Test Port : PMIOPort  Tag=PMCPort  Port=1  Side=Right
  rho : Outport  OutDataType=sfix(16)  OutScaling=2^0
  wires:
  VM/1 -> rho/1
  Drive/1 -> CVS/1
  connections:
  R2/RConn1 -- R3/LConn1 -- CVS/RConn1
  R4/LConn1 -- VM/LConn2 -- R2/LConn1
  G2/LConn1 -- R4/RConn1
  R3/RConn1 -- VM/LConn1 -- Test Port/RConn1
  G1/LConn1 -- CVS/LConn1

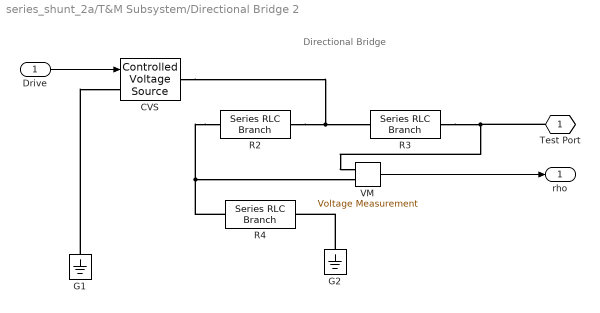
== system series_shunt_2a/T&M Subsystem/Directional Bridge 2 ==
  note: Directional Bridge
  Drive : Inport  OutDataType=sfix(16)  OutScaling=2^0
  CVS : powerlib/Electrical Sources/Controlled Voltage Source  Description=source block  DialogController=POWERSYS.PowerSysDialog  SystemSampleTime=-1  Initialize=off  Source_Type=AC  Amplitude=0  Phase=0  Frequency=0  Measurements=None
      settings: AttributesFormatString=\n
  G1 : powerlib/Elements/Ground  DialogController=POWERSYS.PowerSysDialog  PhysicalDomain=powersysdomain  SubClassName=unknown  LeftPortType=p1  RightPortType=p1  LConnTagsString=a
  G2 : powerlib/Elements/Ground  DialogController=POWERSYS.PowerSysDialog  PhysicalDomain=powersysdomain  SubClassName=unknown  LeftPortType=p1  RightPortType=p1  LConnTagsString=a
  R2 : powerlib/Elements/Series RLC Branch  DialogController=POWERSYS.PowerSysDialog  PhysicalDomain=powersysdomain  SubClassName=unknown  LeftPortType=p1  RightPortType=p1  LConnTagsString=__new0  RConnTagsString=__new0  BranchType=R  Resistance=Zo  Inductance=1.0  SetiL0=off  InitialCurrent=0  Capacitance=1.0  Setx0=off  InitialVoltage=0  Measurements=None
  R3 : powerlib/Elements/Series RLC Branch  DialogController=POWERSYS.PowerSysDialog  PhysicalDomain=powersysdomain  SubClassName=unknown  LeftPortType=p1  RightPortType=p1  LConnTagsString=__new0  RConnTagsString=__new0  BranchType=R  Resistance=Zo  Inductance=1.0  SetiL0=off  InitialCurrent=0  Capacitance=1.0  Setx0=off  InitialVoltage=0  Measurements=None
  R4 : powerlib/Elements/Series RLC Branch  DialogController=POWERSYS.PowerSysDialog  PhysicalDomain=powersysdomain  SubClassName=unknown  LeftPortType=p1  RightPortType=p1  LConnTagsString=__new0  RConnTagsString=__new0  BranchType=R  Resistance=Zo  Inductance=1.0  SetiL0=off  InitialCurrent=0  Capacitance=1.0  Setx0=off  InitialVoltage=0  Measurements=None
  VM : powerlib/Measurements/Voltage Measurement  Tag=PoWeRsYsTeMmEaSuReMeNt  DialogController=POWERSYS.PowerSysDialog  SystemSampleTime=-1  PhasorSimulation=off  OutputType=Magnitude  PSBequivalent=0
  Test Port : PMIOPort  Tag=PMCPort  Port=1  Side=Right
  rho : Outport  OutDataType=sfix(16)  OutScaling=2^0
  wires:
  Drive/1 -> CVS/1
  VM/1 -> rho/1
  connections:
  G1/LConn1 -- CVS/LConn1
  Test Port/RConn1 -- VM/LConn1 -- R3/RConn1
  G2/LConn1 -- R4/RConn1
  R2/LConn1 -- VM/LConn2 -- R4/LConn1
  CVS/RConn1 -- R3/LConn1 -- R2/RConn1

== system series_shunt_2a/T&M Subsystem/Spectrum ==
  Input Signal : Inport  OutDataType=sfix(16)  OutScaling=2^0
  Enable : EnablePort
  Gain : Gain  Gain=1/sqrt(Zo)  ParameterDataType=fixdt(1, 16)  ParameterScaling=2^0  OutDataType=fixdt(1, 16)  OutScaling=2^0
  Spectrum Scope : dspsnks4/Spectrum Scope  DialogController=dspdialog.SpectrumScope  DialogControllerArgs=DataTag12  SystemSampleTime=-1  ScopeProperties=on  Domain=Frequency  HorizSpan=1  UseBuffer=on  BufferSize=512  Overlap=0  inpFftLenInherit=off  FFTlength=128  numAvg=1  DisplayProperties=off  AxisGrid=on  Memory=off  FrameNumber=on  AxisLegend=off  AxisZoom=off  OpenScopeAtSimStart=on  OpenScopeImmediately=off  FigPos=[795 35 408 234]  AxisProperties=off  XUnits=Hertz  XRange=One-sided ([0...Fs/2])  XDisplay=0  InheritXIncr=on  XIncr=1.0  XLabel=Samples  XLimit=Auto  YUnits=dBm  XMax=1  XMin=0  YLabel=dBm  LineProperties=off  wintypeSpecScope=Hann  RsSpecScope=50  betaSpecScope=5  winsampSpecScope=Periodic  XAxisParamsVer=6.9
      settings: YMin=-10  YMax=40
  anti alias : dsparch4/Analog Filter Design  method=Elliptic  filttype=Lowpass  N=8  Wlo=BW*2*pi  Whi=80  Rp=0.11  Rs=100
  sampler : ZeroOrderHold  SampleTime=1/(2.56*BW)
  wires:
  sampler/1 -> Gain/1
  anti alias/1 -> sampler/1
  Input Signal/1 -> anti alias/1
  Gain/1 -> Spectrum Scope/1

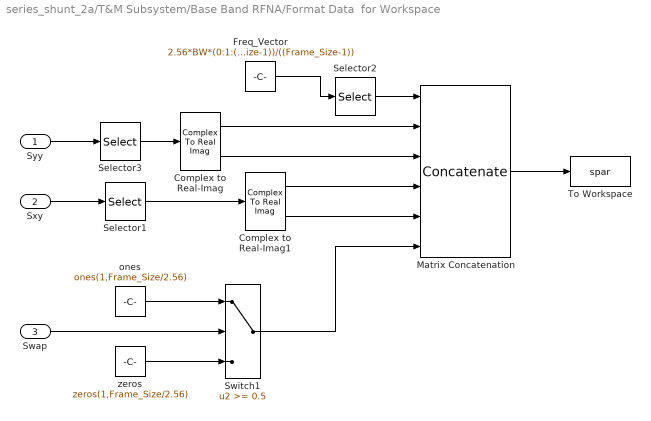
== system series_shunt_2a/T&M Subsystem/Base Band RFNA/Format Data  for Workspace ==
  Syy : Inport  OutDataType=sfix(16)  OutScaling=2^0
  Sxy : Inport  Port=2  OutDataType=sfix(16)  OutScaling=2^0
  Swap : Inport  Port=3  OutDataType=sfix(16)  OutScaling=2^0
  Complex to Real-Imag : ComplexToRealImag
  Complex to Real-Imag1 : ComplexToRealImag
  Freq_Vector : Constant  Value=2.56*BW*(0:1:(Frame_Size-1))/((Frame_Size-1))  OutDataType=sfix(16)  OutScaling=2^0
  Matrix Concatenation : Concatenate  NumInputs=6  Mode=Multidimensional array  ConcatenateDimension=2
  Selector1 : Selector  InputPortWidth=Frame_Size  IndexOptions=Index vector (dialog)  Indices=[1:Frame_Size/2.56]  OutputSizes=1
  Selector2 : Selector  InputPortWidth=Frame_Size  IndexOptions=Index vector (dialog)  Indices=[1:Frame_Size/2.56]  OutputSizes=1
  Selector3 : Selector  InputPortWidth=Frame_Size  IndexOptions=Index vector (dialog)  Indices=[1:Frame_Size/2.56]  OutputSizes=1
  Switch1 : Switch  Threshold=0.5  SaturateOnIntegerOverflow=on
  To Workspace : ToWorkspace  VariableName=spar  SampleTime=-1  SaveFormat=Array
      settings: MaxDataPoints=1
  ones : Constant  Value=ones(1,Frame_Size/2.56)  OutDataType=sfix(16)  OutScaling=2^0
  zeros : Constant  Value=zeros(1,Frame_Size/2.56)  OutDataType=sfix(16)  OutScaling=2^0
  wires:
  Matrix Concatenation/1 -> To Workspace/1
  Complex to Real-Imag1/2 -> Matrix Concatenation/5
  Freq_Vector/1 -> Selector2/1
  Complex to Real-Imag/1 -> Matrix Concatenation/2
  Complex to Real-Imag/2 -> Matrix Concatenation/3
  Complex to Real-Imag1/1 -> Matrix Concatenation/4
  Syy/1 -> Selector3/1
  Sxy/1 -> Selector1/1
  ones/1 -> Switch1/1
  zeros/1 -> Switch1/3
  Swap/1 -> Switch1/2
  Switch1/1 -> Matrix Concatenation/6
  Selector3/1 -> Complex to Real-Imag/1
  Selector1/1 -> Complex to Real-Imag1/1
  Selector2/1 -> Matrix Concatenation/1

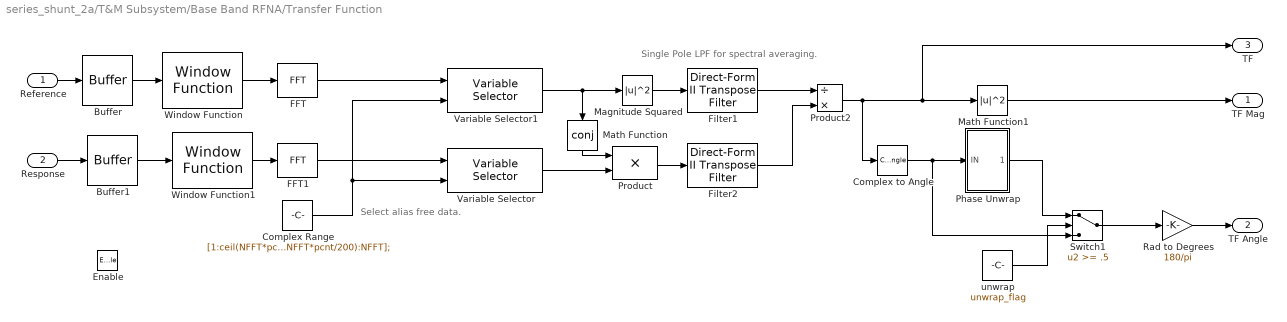
== system series_shunt_2a/T&M Subsystem/Base Band RFNA/Transfer Function  ==
  note: Select alias free data.
  note: Single Pole LPF for spectral averaging.
  Reference : Inport  OutDataType=sfix(16)  OutScaling=2^0
  Response : Inport  Port=2  OutDataType=sfix(16)  OutScaling=2^0
  Enable : EnablePort
  Buffer : dspbuff3/Buffer  N=NFFT  V=0  ic=0
  Buffer1 : dspbuff3/Buffer  N=NFFT  V=0  ic=0
  Complex Range : Constant  Value=[1:ceil(NFFT*pcnt/200),ceil(1+NFFT-NFFT*pcnt/200):NFFT];  OutDataType=sfix(16)  OutScaling=2^0
  Complex to Angle : ComplexToMagnitudeAngle  Output=Angle
  FFT : dspxfrm3/FFT  DialogController=dspDDGCreate  DialogControllerArgs=DataTag2  CompMethod=Table lookup  TableOpt=NEW  TableOptActive=Speed  BitRevOrder=off  InheritFFTLength=on  FFTLength=64  SkipNorm=on  firstCoeffMode=Specify word length  firstCoeffWordLength=16  firstCoeffFracLength=15  roundingMode=Floor  overflowMode=off
  FFT1 : dspxfrm3/FFT  DialogController=dspDDGCreate  DialogControllerArgs=DataTag3  CompMethod=Table lookup  TableOpt=NEW  TableOptActive=Speed  BitRevOrder=off  InheritFFTLength=on  FFTLength=64  SkipNorm=on  firstCoeffMode=User-defined  firstCoeffWordLength=16  firstCoeffFracLength=15  roundingMode=Floor  overflowMode=off
  Filter1 : dsparch3/Direct-Form II Transpose Filter  num=1  den=[Navg -(Navg-1)]  ic=eps
  Filter2 : dsparch3/Direct-Form II Transpose Filter  num=1  den=[Navg -(Navg-1)]  ic=eps
  Magnitude Squared : Math  Operator=magnitude^2  OutDataType=sfix(16)  OutScaling=2^0  SaturateOnIntegerOverflow=on
  Math Function : Math  Operator=conj  OutDataType=sfix(16)  OutScaling=2^0  SaturateOnIntegerOverflow=on
  Math Function1 : Math  Operator=magnitude^2  OutDataType=sfix(16)  OutScaling=2^0  SaturateOnIntegerOverflow=on
  Phase Unwrap : Subsystem
  Product : Product  OutDataType=sfix(16)  OutScaling=2^0  SaturateOnIntegerOverflow=on  InputSameDT=on  OutDataTypeStr=Inherit: Same as first input
  Product2 : Product  Inputs=/*  OutDataType=sfix(16)  OutScaling=2^0  SaturateOnIntegerOverflow=on  InputSameDT=on  OutDataTypeStr=Inherit: Same as first input
  Rad to Degrees : Gain  Gain=180/pi  ParameterDataType=sfix(16)  ParameterScaling=2^0  OutDataType=sfix(16)  OutScaling=2^0
  Switch1 : Switch  Threshold=.5
  Variable Selector : dspindex/Variable Selector  NumInputs=1  rowsOrCols=Rows  IdxMode=Variable  Elements=[1 3]  ZerOneIdxMode=One-based  errmode=Clip Index  FillMode=on  FillValues=0
  Variable Selector1 : dspindex/Variable Selector  NumInputs=1  rowsOrCols=Rows  IdxMode=Variable  Elements=[1 3]  ZerOneIdxMode=One-based  errmode=Clip Index  FillMode=on  FillValues=0
  Window Function : dspsigops/Window Function  DialogController=dspDDGCreate  DialogControllerArgs=DataTag5  winmode=Apply window to input  wintype=Hann  sampmode=Continuous  samptime=1  N=64  Rs=50  beta=10  winsamp=Periodic  UserWindow=hamming  OptParams=off  UserParams={'symmetric'}  dataType=double  isSigned=on  wordLen=16  udDataType=sfix(16)  fracBitsMode=Best precision  numFracBits=15  roundingMode=Floor  overflowMode=off  numSidelobes=4  sidelobeLevel=-30
  Window Function1 : dspsigops/Window Function  DialogController=dspDDGCreate  DialogControllerArgs=DataTag6  winmode=Apply window to input  wintype=Hann  sampmode=Continuous  samptime=1  N=64  Rs=50  beta=10  winsamp=Periodic  UserWindow=hamming  OptParams=off  UserParams={'symmetric'}  dataType=double  isSigned=on  wordLen=16  udDataType=sfix(16)  fracBitsMode=Best precision  numFracBits=15  roundingMode=Floor  overflowMode=off  numSidelobes=4  sidelobeLevel=-30
  unwrap : Constant  Value=unwrap_flag  OutDataType=sfix(16)  OutScaling=2^0
  TF Mag : Outport  OutDataType=sfix(16)  OutScaling=2^0
  TF Angle : Outport  Port=2  OutDataType=sfix(16)  OutScaling=2^0
  "TF " : Outport  Port=3  OutDataType=sfix(16)  OutScaling=2^0
  wires:
  Phase Unwrap/1(Out1) -> Switch1/1
  unwrap/1 -> Switch1/2
  Switch1/1 -> Rad to Degrees/1
  Variable Selector1/1 -> Math Function/1, Magnitude Squared/1
  Variable Selector/1 -> Product/2
  Product2/1 -> Complex to Angle/1, Math Function1/1, "TF "/1
  Buffer1/1 -> Window Function1/1
  Buffer/1 -> Window Function/1
  Filter2/1 -> Product2/2
  Filter1/1 -> Product2/1
  Window Function1/1 -> FFT1/1
  Window Function/1 -> FFT/1
  Math Function1/1 -> TF Mag/1
  FFT/1 -> Variable Selector1/1
  Magnitude Squared/1 -> Filter1/1
  Math Function/1 -> Product/1
  FFT1/1 -> Variable Selector/1
  Product/1 -> Filter2/1
  Reference/1 -> Buffer/1
  Response/1 -> Buffer1/1
  Rad to Degrees/1 -> TF Angle/1
  Complex to Angle/1 -> Phase Unwrap/1(IN), Switch1/3
  Complex Range/1 -> Variable Selector1/2, Variable Selector/2

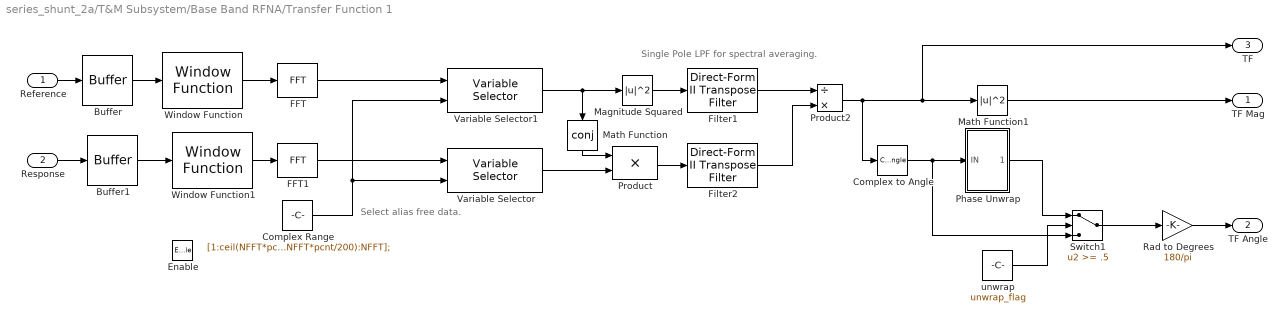
== system series_shunt_2a/T&M Subsystem/Base Band RFNA/Transfer Function 1 ==
  note: Single Pole LPF for spectral averaging.
  note: Select alias free data.
  Reference : Inport  OutDataType=sfix(16)  OutScaling=2^0
  Response : Inport  Port=2  OutDataType=sfix(16)  OutScaling=2^0
  Enable : EnablePort
  Buffer : dspbuff3/Buffer  N=NFFT  V=0  ic=0
  Buffer1 : dspbuff3/Buffer  N=NFFT  V=0  ic=0
  Complex Range : Constant  Value=[1:ceil(NFFT*pcnt/200),ceil(1+NFFT-NFFT*pcnt/200):NFFT];  OutDataType=sfix(16)  OutScaling=2^0
  Complex to Angle : ComplexToMagnitudeAngle  Output=Angle
  FFT : dspxfrm3/FFT  DialogController=dspDDGCreate  DialogControllerArgs=DataTag7  CompMethod=Table lookup  TableOpt=NEW  TableOptActive=Speed  BitRevOrder=off  InheritFFTLength=on  FFTLength=64  SkipNorm=on  firstCoeffMode=Specify word length  firstCoeffWordLength=16  firstCoeffFracLength=15  roundingMode=Floor  overflowMode=off
  FFT1 : dspxfrm3/FFT  DialogController=dspDDGCreate  DialogControllerArgs=DataTag8  CompMethod=Table lookup  TableOpt=NEW  TableOptActive=Speed  BitRevOrder=off  InheritFFTLength=on  FFTLength=64  SkipNorm=on  firstCoeffMode=User-defined  firstCoeffWordLength=16  firstCoeffFracLength=15  roundingMode=Floor  overflowMode=off
  Filter1 : dsparch3/Direct-Form II Transpose Filter  num=1  den=[Navg -(Navg-1)]  ic=eps
  Filter2 : dsparch3/Direct-Form II Transpose Filter  num=1  den=[Navg -(Navg-1)]  ic=eps
  Magnitude Squared : Math  Operator=magnitude^2  OutDataType=sfix(16)  OutScaling=2^0  SaturateOnIntegerOverflow=on
  Math Function : Math  Operator=conj  OutDataType=sfix(16)  OutScaling=2^0  SaturateOnIntegerOverflow=on
  Math Function1 : Math  Operator=magnitude^2  OutDataType=sfix(16)  OutScaling=2^0  SaturateOnIntegerOverflow=on
  Phase Unwrap : Subsystem
  Product : Product  OutDataType=sfix(16)  OutScaling=2^0  SaturateOnIntegerOverflow=on  InputSameDT=on  OutDataTypeStr=Inherit: Same as first input
  Product2 : Product  Inputs=/*  OutDataType=sfix(16)  OutScaling=2^0  SaturateOnIntegerOverflow=on  InputSameDT=on  OutDataTypeStr=Inherit: Same as first input
  Rad to Degrees : Gain  Gain=180/pi  ParameterDataType=sfix(16)  ParameterScaling=2^0  OutDataType=sfix(16)  OutScaling=2^0
  Switch1 : Switch  Threshold=.5
  Variable Selector : dspindex/Variable Selector  NumInputs=1  rowsOrCols=Rows  IdxMode=Variable  Elements=[1 3]  ZerOneIdxMode=One-based  errmode=Clip Index  FillMode=on  FillValues=0
  Variable Selector1 : dspindex/Variable Selector  NumInputs=1  rowsOrCols=Rows  IdxMode=Variable  Elements=[1 3]  ZerOneIdxMode=One-based  errmode=Clip Index  FillMode=on  FillValues=0
  Window Function : dspsigops/Window Function  DialogController=dspDDGCreate  DialogControllerArgs=DataTag10  winmode=Apply window to input  wintype=Hann  sampmode=Continuous  samptime=1  N=64  Rs=50  beta=10  winsamp=Periodic  UserWindow=hamming  OptParams=off  UserParams={'symmetric'}  dataType=double  isSigned=on  wordLen=16  udDataType=sfix(16)  fracBitsMode=Best precision  numFracBits=15  roundingMode=Floor  overflowMode=off  numSidelobes=4  sidelobeLevel=-30
  Window Function1 : dspsigops/Window Function  DialogController=dspDDGCreate  DialogControllerArgs=DataTag11  winmode=Apply window to input  wintype=Hann  sampmode=Continuous  samptime=1  N=64  Rs=50  beta=10  winsamp=Periodic  UserWindow=hamming  OptParams=off  UserParams={'symmetric'}  dataType=double  isSigned=on  wordLen=16  udDataType=sfix(16)  fracBitsMode=Best precision  numFracBits=15  roundingMode=Floor  overflowMode=off  numSidelobes=4  sidelobeLevel=-30
  unwrap : Constant  Value=unwrap_flag  OutDataType=sfix(16)  OutScaling=2^0
  TF Mag : Outport  OutDataType=sfix(16)  OutScaling=2^0
  TF Angle : Outport  Port=2  OutDataType=sfix(16)  OutScaling=2^0
  "TF " : Outport  Port=3  OutDataType=sfix(16)  OutScaling=2^0
  wires:
  Complex Range/1 -> Variable Selector/2, Variable Selector1/2
  Complex to Angle/1 -> Switch1/3, Phase Unwrap/1(IN)
  Rad to Degrees/1 -> TF Angle/1
  Response/1 -> Buffer1/1
  Reference/1 -> Buffer/1
  Product/1 -> Filter2/1
  FFT1/1 -> Variable Selector/1
  Math Function/1 -> Product/1
  Magnitude Squared/1 -> Filter1/1
  FFT/1 -> Variable Selector1/1
  Math Function1/1 -> TF Mag/1
  Window Function/1 -> FFT/1
  Window Function1/1 -> FFT1/1
  Filter1/1 -> Product2/1
  Filter2/1 -> Product2/2
  Buffer/1 -> Window Function/1
  Buffer1/1 -> Window Function1/1
  Product2/1 -> "TF "/1, Math Function1/1, Complex to Angle/1
  Variable Selector/1 -> Product/2
  Variable Selector1/1 -> Magnitude Squared/1, Math Function/1
  Switch1/1 -> Rad to Degrees/1
  unwrap/1 -> Switch1/2
  Phase Unwrap/1(Out1) -> Switch1/1

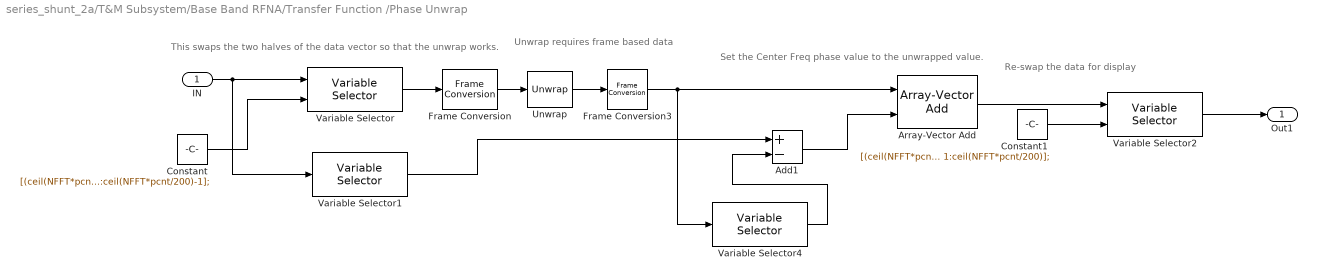
== system series_shunt_2a/T&M Subsystem/Base Band RFNA/Transfer Function /Phase Unwrap ==
  note: Unwrap requires frame based data
  note: Re-swap the data for display
  note: Set the Center Freq phase value to the unwrapped value.
  note: This swaps the two halves of the data vector
      | so that the unwrap works.
  IN : Inport  OutDataType=sfix(16)  OutScaling=2^0
  Add1 : Sum  Inputs=+-  OutDataType=sfix(16)  OutScaling=2^-10
  Array-Vector Add : dspmtrx3/Array-Vector Add  DialogController=dspDDGCreate  DialogControllerArgs=DataTag4  Dimension=2  V_Source=Input port  V_VectFromMask=[0.5 0.25]  firstCoeffDataTypeStr=Inherit: Same word length as input  firstCoeffLastDataTypeStr=Inherit: Same word length as input  firstCoeffMin=[]  firstCoeffMax=[]  outputDataTypeStr=Inherit: Same as accumulator  outputLastDataTypeStr=Inherit: Same as accumulator  outputMin=[]  outputMax=[]  roundingMode=Floor  overflowMode=off
  Constant : Constant  Value=[(ceil(NFFT*pcnt/200)):ceil(NFFT*pcnt/100) 1:ceil(NFFT*pcnt/200)-1];  OutDataType=sfix(16)  OutScaling=2^0
  Constant1 : Constant  Value=[(ceil(NFFT*pcnt/200)+1):ceil(NFFT*pcnt/100) 1:ceil(NFFT*pcnt/200)];  OutDataType=sfix(16)  OutScaling=2^0
  Frame Conversion : FrameConversion
  Frame Conversion3 : FrameConversion  OutFrame=Sample-based
  Unwrap : dspsigops/Unwrap  running=on  tol=pi
  Variable Selector : dspindex/Variable Selector  NumInputs=1  rowsOrCols=Rows  IdxMode=Variable  Elements=[1 3]  ZerOneIdxMode=One-based  errmode=Clip Index  FillMode=on  FillValues=0
  Variable Selector1 : dspindex/Variable Selector  NumInputs=1  rowsOrCols=Rows  IdxMode=Fixed  Elements=[1]  ZerOneIdxMode=One-based  errmode=Clip Index  FillMode=on  FillValues=0
  Variable Selector2 : dspindex/Variable Selector  NumInputs=1  rowsOrCols=Rows  IdxMode=Variable  Elements=[1 3]  ZerOneIdxMode=One-based  errmode=Clip Index  FillMode=on  FillValues=0
  Variable Selector4 : dspindex/Variable Selector  NumInputs=1  rowsOrCols=Rows  IdxMode=Fixed  Elements=length([(ceil(NFFT*pcnt/200)+1):ceil(NFFT*pcnt/100) 1:ceil(NFFT*pcnt/200)] )/2+1  ZerOneIdxMode=One-based  errmode=Clip Index  FillMode=on  FillValues=0
  Out1 : Outport  OutDataType=sfix(16)  OutScaling=2^0
  wires:
  Array-Vector Add/1 -> Variable Selector2/1
  Add1/1 -> Array-Vector Add/2
  Frame Conversion3/1 -> Array-Vector Add/1, Variable Selector4/1
  Constant1/1 -> Variable Selector2/2
  Variable Selector4/1 -> Add1/2
  Unwrap/1 -> Frame Conversion3/1
  Variable Selector1/1 -> Add1/1
  Variable Selector/1 -> Frame Conversion/1
  Constant/1 -> Variable Selector/2
  IN/1 -> Variable Selector1/1, Variable Selector/1
  Variable Selector2/1 -> Out1/1
  Frame Conversion/1 -> Unwrap/1
